simulink model "main_adaptive"  (R2016b)
settings: Solver=VariableStepAuto  StartTime=0.0  StopTime=0.2  FixedStep=2e-4  RelTol=1e-3
values from neighbouring files (symbols this model uses):
  adaptiveFIRCoef = adaptiveFIRCoef+R*(y-phi'*adaptiveFIRCoef)/lambda    [adaptiveLaw.m]    (also in adaptiveLawWithConstraint.m; initiateSimulation.m = zeros(firOrder,1))
  F1 = numGpDis/sum(numGpDis)    [initiateSimulation.m]
  F2 = denGpDis/sum(numGpDis)    [initiateSimulation.m]
  fs = 5000    [initiateSimulation.m]
  Ts = 1/fs    (= 0.0002)    [initiateSimulation.m]
  TsN = 1e-5    (= 1e-05)    [initiateSimulation.m]
undefined symbols (not defined in the file or in its folder): denGcDis, denGp, denIIR, numGcDis, numGp, numIIR
libraries: simulink x3, model_controller x1
settings Model: Creator=Dai Luyao  LastModifiedBy=Dai Luyao

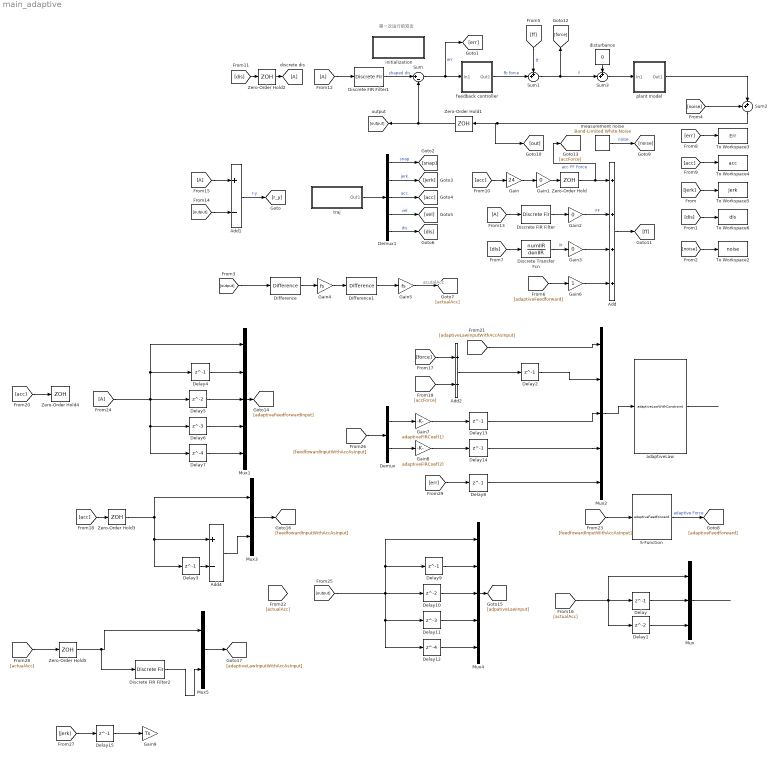
== system main_adaptive ==
  note: acutalAcc
  note: 第一次运行前双击
  Add : Sum  Inputs=++++
  Add1 : Sum  Inputs=+-
  Add2 : Sum  Inputs=+-
  Add4 : Sum  Inputs=+-
  Delay{,2..3,8,13..15} (7 alike) : Delay  DelayLength=1  SampleTime=Ts
  Delay1 : Delay  SampleTime=Ts
  Delay10 : Delay
  Delay11 : Delay  DelayLength=3
  Delay12 : Delay  DelayLength=4
  Delay4 : Delay  DelayLength=1
  Delay5 : Delay
  Delay6 : Delay  DelayLength=3
  Delay7 : Delay  DelayLength=4
  Delay9 : Delay  DelayLength=1
  Demux : Demux  Outputs=2
  Demux1 : Demux  Outputs=5
  Difference : simulink/Discrete/Difference  ICPrevInput=0.0  OutMin=[]  OutMax=[]  OutDataType=fixdt(1, 16)  OutScaling=2^-10  DoSatur=off
  Difference1 : simulink/Discrete/Difference  ICPrevInput=0.0  OutMin=[]  OutMax=[]  OutDataType=fixdt(1, 16)  OutScaling=2^-10  DoSatur=off
  Discrete Transfer Fcn : DiscreteTransferFcn  Numerator=numIIR  Denominator=denIIR  SampleTime=Ts
  Discrete FIR Filter : DiscreteFir  Coefficients=F2  SampleTime=Ts
  Discrete FIR Filter1 : DiscreteFir  Coefficients=F1  SampleTime=Ts
  Discrete FIR Filter2 : DiscreteFir  Coefficients=[1 -1]  SampleTime=Ts
  Gain : Gain  Gain=24
  Gain1 : Gain  Gain=0
  Gain2 : Gain  Gain=0
  Gain3 : Gain  Gain=0
  Gain4 : Gain  Gain=fs
  Gain5 : Gain  Gain=fs
  Gain6 : Gain
  Gain7 : Gain  Gain=adaptiveFIRCoef(1)
  Gain8 : Gain  Gain=adaptiveFIRCoef(2)
  Gain9 : Gain  Gain=Ts
  Mux : Mux  Inputs=3
  Mux1 : Mux  Inputs=5
  Mux2 : Mux  Inputs=5
  Mux3 : Mux  Inputs=2
  Mux4 : Mux  Inputs=5
  Mux5 : Mux  Inputs=2
  S-Function : S-Function  FunctionName=adaptiveFeedforward  SFunctionDeploymentMode=off  EnableBusSupport=off
  Sum : Sum  Inputs=|+-
  Sum1 : Sum  Inputs=++|
  Sum2 : Sum  Inputs=++|
  Sum3 : Sum  Inputs=++|
  To Workspace2 : ToWorkspace  VariableName=noise  SaveFormat=Structure With Time  SampleTime=-1
  To Workspace3 : ToWorkspace  VariableName=Err  SaveFormat=Structure With Time  SampleTime=-1
  To Workspace4 : ToWorkspace  VariableName=acc  SaveFormat=Structure With Time  SampleTime=-1
  To Workspace5 : ToWorkspace  VariableName=jerk  SaveFormat=Structure With Time  SampleTime=-1
  To Workspace6 : ToWorkspace  VariableName=dis  SaveFormat=Structure With Time  SampleTime=-1
  Zero-Order Hold{,1..5} (6 alike) : ZeroOrderHold  SampleTime=Ts
  adaptiveLaw : S-Function  FunctionName=adaptiveLawWithConstraint  SFunctionDeploymentMode=off  EnableBusSupport=off
  disturbance : Constant  Value=0
  feedback controller : Subsystem
  initialization : Subsystem
      settings: OpenFcn=initiateSimulation;  MoveFcn=edit initiateSimulation;
  measurement noise : simulink/Sources/Band-Limited White Noise  Cov=noisePower  Ts=TsN  seed=[23341]
  plant model : Subsystem
  traj : Subsystem  BlockChoice=4th order traj
      link override 3rd order traj: j=800  v=0.25  x=0.06  a=10
      link override 4th order traj: a=10  v=0.25  x=0.05  j=800  d=64000
      settings: AttributesFormatString=%<BlockChoice>  TemplateBlock=model_controller/Profile Generators/traj  MemberBlocks=2nd order traj,3rd order traj,4th order traj,step,zero
  wires:
  Sum/1 -> feedback controller/1(In1), [err]  "err"
  Sum1/1 -> Sum3/2, [force]  "f"
  measurement noise/1 -> [noise]  "noise"
  Demux1/1 -> [snap]  "snap"
  Demux1/2 -> [jerk]  "jerk"
  Demux1/3 -> [acc]  "acc"
  Demux1/4 -> [vel]  "vel"
  Demux1/5 -> [dis]  "dis"
  [acc] -> To Workspace4/1
  [acc] -> Gain/1
  [jerk] -> To Workspace5/1
  traj/1(Out1) -> Demux1/1
  [ff] -> Sum1/1  "ff"
  [dis] -> To Workspace6/1
  [err] -> To Workspace3/1
  [noise] -> To Workspace2/1
  disturbance/1 -> Sum3/1
  Sum3/1 -> plant model/1(In1)
  plant model/1(Out1) -> Sum2/2
  Discrete FIR Filter/1 -> Gain2/1
  Add/1 -> [ff]
  Sum2/1 -> Zero-Order Hold1/1, [out]
  Gain/1 -> Gain1/1
  feedback controller/1(Out1) -> Sum1/2  "fb force"
  Gain2/1 -> Add/2  "FF"
  Discrete Transfer Fcn/1 -> Gain3/1  "iir"
  Gain3/1 -> Add/3
  [dis] -> Discrete Transfer Fcn/1
  Gain1/1 -> Zero-Order Hold/1
  Zero-Order Hold/1 -> [accForce], Add/1  "acc FF Force"
  Discrete FIR Filter1/1 -> Sum/1  "shaped dis"
  Zero-Order Hold1/1 -> Sum/2, [output]
  [dis] -> Zero-Order Hold2/1
  Zero-Order Hold2/1 -> [A]
  [A] -> Discrete FIR Filter1/1
  [A] -> Discrete FIR Filter/1
  [output] -> Add1/2
  [A] -> Add1/1
  Add1/1 -> [r_y]  "r-y"
  [output] -> Difference/1
  Difference1/1 -> Gain5/1
  Gain4/1 -> Difference1/1
  Difference/1 -> Gain4/1
  Gain5/1 -> [actualAcc]
  [adaptiveFeedforward] -> Gain6/1
  Gain6/1 -> Add/4
  Delay4/1 -> Mux1/2
  Delay5/1 -> Mux1/3
  Delay6/1 -> Mux1/4
  Delay7/1 -> Mux1/5
  Mux2/1 -> adaptiveLaw/1
  S-Function/1 -> [adaptiveFeedforward]  "adaptive Force"
  [force] -> Add2/1
  [accForce] -> Add2/2
  adaptiveLaw/1 -> ?
  Mux3/1 -> [feedfowardInputWithAccAsInput]
  [acc] -> Zero-Order Hold3/1
  Zero-Order Hold3/1 -> Mux3/1, Add4/1, Delay3/1
  Mux1/1 -> [adaptiveFeedforwardInput]
  [feedfowardInputWithAccAsInput] -> S-Function/1
  Delay9/1 -> Mux4/2
  Delay10/1 -> Mux4/3
  Delay11/1 -> Mux4/4
  Delay12/1 -> Mux4/5
  Mux4/1 -> [adpativeLawInput]
  [actualAcc] -> Mux/1, Delay/1, Delay1/1
  Delay1/1 -> Mux/3
  Delay/1 -> Mux/2
  Mux/1 -> ?
  [adaptiveLawInputWithAccAsInput] -> Mux2/1
  [acc] -> Zero-Order Hold4/1
  [A] -> Delay7/1, Delay6/1, Mux1/1, Delay4/1, Delay5/1
  [output] -> Delay12/1, Delay11/1, Mux4/1, Delay9/1, Delay10/1
  Delay3/1 -> Add4/2
  Add4/1 -> Mux3/2
  Mux5/1 -> [adaptiveLawInputWithAccAsInput]
  [actualAcc] -> Zero-Order Hold5/1
  Zero-Order Hold5/1 -> Discrete FIR Filter2/1, Mux5/1
  Add2/1 -> Delay2/1
  Delay2/1 -> Mux2/2
  [feedfowardInputWithAccAsInput] -> Demux/1
  Demux/1 -> Gain7/1
  Demux/2 -> Gain8/1
  Gain7/1 -> Delay13/1
  Gain8/1 -> Delay14/1
  Delay13/1 -> Mux2/3
  Delay14/1 -> Mux2/4
  [jerk] -> Delay15/1
  [noise] -> Sum2/1
  Delay15/1 -> Gain9/1
  [err] -> Delay8/1
  Delay8/1 -> Mux2/5
  Discrete FIR Filter2/1 -> Mux5/2

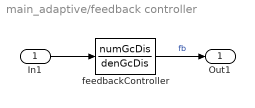
== system main_adaptive/feedback controller ==
  In1 : Inport
  feedbackController : DiscreteTransferFcn  Numerator=numGcDis  Denominator=denGcDis  SampleTime=Ts
  Out1 : Outport
  wires:
  feedbackController/1 -> Out1/1  "fb"
  In1/1 -> feedbackController/1

== system main_adaptive/initialization ==

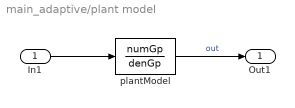
== system main_adaptive/plant model ==
  In1 : Inport
  plantModel : TransferFcn  Numerator=numGp  Denominator=denGp
  Out1 : Outport
  wires:
  In1/1 -> plantModel/1
  plantModel/1 -> Out1/1  "out"

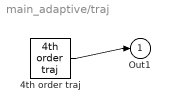
== system main_adaptive/traj ==
  4th order traj : model_controller/Profile Generators/4th order traj  t0=0  x=0.05  v=0.25  a=10  j=800  d=64000  Ts=0
  Out1 : Outport
  wires:
  4th order traj/1 -> Out1/1
